simulink model "PV_grid_connected_Inverter"  (R2022b)
settings: Solver=ode23tb  StartTime=0.0  StopTime=2  FixedStep=Ts_Power  RelTol=1e-4
PreLoadFcn:
  | Ts_Power=50e-6;
  | Ts_Control=100e-6;
InitFcn:
  | Ts_Power=50e-6;
  | Ts_Control=100e-6;
undefined symbols (not defined in the file): sigbuilder_block
libraries: spsIGBTDiodeLib x7, spsSeriesRLCBranchLib x3, spsThreePhaseSeriesRLCBranchLib x1, spsThreePhaseSourceLib x1, slpidlib x1, spsPLL3phLib x1, spsabctodq0Lib x1, spsdq0toabcLib x1, spsDiodeLib x1, spsGroundLib x1, spsMeanLib x1, spsPower3phInstantaneousLib x1
Description:
  | Copyright 2008-2017 The MathWorks, Inc.
settings Model: Creator=MathWorks  LastModifiedBy=mohua
settings SolverCC: SolverJacobianMethodControl=FullAnalytical  ZeroCrossAlgorithm=Adaptive  AlgebraicLoopSolver=TrustRegion
settings DataIOCC: LimitDataPoints=on  SaveFormat=Array  SignalLoggingSaveFormat=ModelDataLogs  ReturnWorkspaceOutputs=off
settings OptimizationCC: ExpressionDepthLimit=2147483647  LifeSpan=inf
settings DebuggingCC: UnderspecifiedInitializationDetection=Classic  MergeDetectMultiDrivingBlocksExec=none  SolverPrmCheckMsg=warning  FcnCallInpInsideContextMsg=warning  UnconnectedInputMsg=warning  UnconnectedOutputMsg=warning  UnconnectedLineMsg=warning  StateNameClashWarn=warning  SFUnexpectedBacktrackingDiag=warning  SFNoUnconditionalDefaultTransitionDiag=warning  SFExecutionAtInitializationDiag=none  SFMachineParentedDataDiag=warning  ArithmeticOperatorsInVariantConditions=warning
settings HardwareCC: ProdBitPerPointer=32  ProdBitPerSizeT=32  ProdBitPerPtrDiffT=32  ProdLargestAtomicFloat=None  ProdIntDivRoundTo=Undefined  ProdEndianess=Unspecified  ProdWordSize=32  ProdHWDeviceType=32-bit Generic
settings ModelReferenceCC: EnableRefExpFcnMdlSchedulingChecks=on  PropagateSignalLabelsOutOfModel=off
settings SFSimCC: SimUseLocalCustomCode=off  CustomCodeUndefinedFunction=UseInterfaceOnly
settings RTWCC: RTWUseLocalCustomCode=off
settings CodeAppCC: StateflowObjectComments=on
settings GRTTargetCC: TargetLangStandard=C89/C90 (ANSI)  CombineOutputUpdateFcns=off  GRTInterface=on
settings ConfigComp: CovMetricSettings=dw  CovSaveCumulativeToWorkspaceVar=on  CovSaveSingleToWorkspaceVar=on  CovExternalEMLEnable=off  CovSFcnEnable=off
settings SimscapeCC: SimscapeNormalizeSystem=off

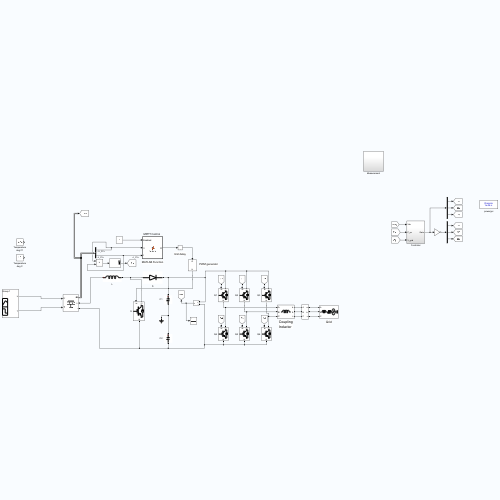
[thumbnail: Simulink's stored preview of the top-level diagram]
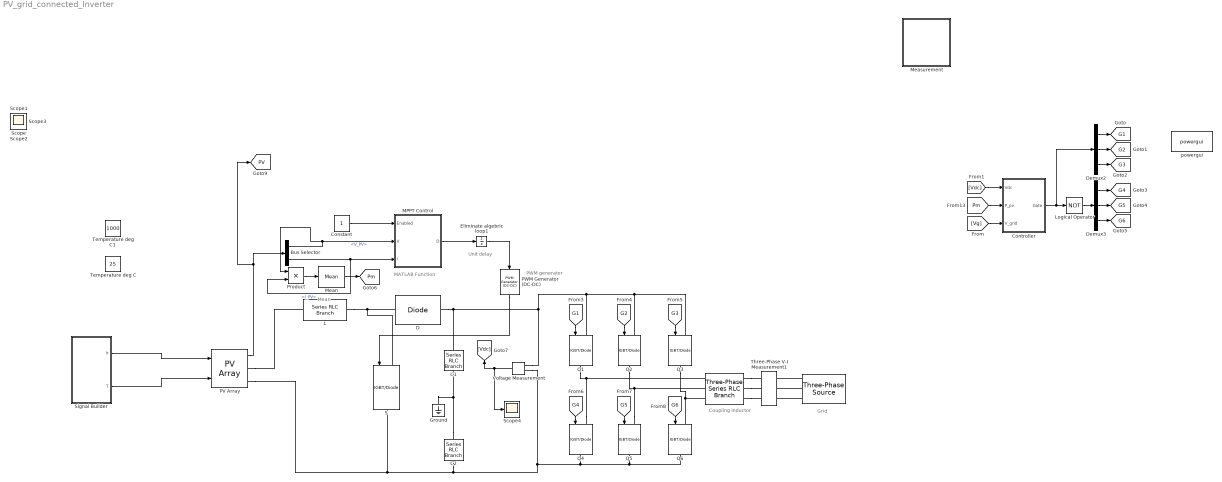
== system PV_grid_connected_Inverter ==
  note: Grid
  note: Coupling
      | Inductor
  note: MATLAB Function
  note: Mean
  note: PWM generator
  note: Unit delay
  " " : spsThreePhaseSeriesRLCBranchLib/Three-Phase Series RLC Branch  LConnTagsString=A|B|C  RConnTagsString=A|B|C  BranchType=L  Resistance=0.09  Inductance=0.28e-3  Capacitance=1e-6  Measurements=None
  "  " : spsThreePhaseSourceLib/Three-Phase Source  InternalConnection=Yg  VoltagePhases=off  Voltage=400  PhaseAngle=0  Voltage_phases=[25e3 25e3 25e3]/sqrt(3)  PhaseAngles_phases=[0 -120 +120]  Frequency=50  NonIdealSource=on  SpecifyImpedance=on  Resistance=0.8929  Inductance=16.58e-3  ShortCircuitLevel=100e6  BaseVoltage=400  XRratio=10  BusType=swing  Pref=0  Qref=0  Prefabc=[10e3, 10e3, 10e3]  Qrefabc=[0, 0, 0]  Qmin=-inf  Qmax=inf
  Bus Selector : BusSelector  OutputSignals=V_PV,I_PV
  C1 : spsSeriesRLCBranchLib/Series RLC Branch  LConnTagsString=__new0  RConnTagsString=__new0  BranchType=C  Resistance=1  Inductance=1e-3  SetiL0=off  InitialCurrent=0  Capacitance=4700e-6  Setx0=on  InitialVoltage=350  Measurements=None
  C2 : spsSeriesRLCBranchLib/Series RLC Branch  LConnTagsString=__new0  RConnTagsString=__new0  BranchType=C  Resistance=1  Inductance=1e-3  SetiL0=off  InitialCurrent=0  Capacitance=4700e-6  Setx0=on  InitialVoltage=350  Measurements=None
  Constant : Constant
  Controller : Subsystem
  D : spsDiodeLib/Diode  Ron=0.001  Lon=0  Vf=0.8  IC=0  UseSnubber=0  Rs=inf  Cs=250e-9  Measurements=off
  Demux2 : Demux  Outputs=3
  Demux3 : Demux  Outputs=3
  Eliminate algebric loop1 : UnitDelay  InitialCondition=0.485  SampleTime=Ts_Control  HasFrameUpgradeWarning=on
  Ground : spsGroundLib/Ground  LConnTagsString=a
  L : spsSeriesRLCBranchLib/Series RLC Branch  LConnTagsString=__new0  RConnTagsString=__new0  BranchType=L  Resistance=0.001  Inductance=4e-3  SetiL0=off  InitialCurrent=0  Capacitance=1e-6  Setx0=off  InitialVoltage=0  Measurements=None
  Logical Operator : Logic  Operator=NOT  IconShape=distinctive  AllPortsSameDT=off  OutDataTypeStr=boolean
  "MPPT Control  " : MATLAB Function  TreatAsAtomicUnit=on
  Mean : spsMeanLib/Mean  Freq=50  Vinit=0  Ts=0
  Measurement : Subsystem
  PV Array : spsPVArrayLib/PV Array  Npar=64  Nser=5  PlotType=array @ 1000 W/m2 & specified temperatures  S_vec="[ 1000  500  100 ]"  Temp_C_vec="[ 45 25  ]"  ModuleName=SunPower SPR-315E-WHT-D  PlotWhenSelected=off  Pm=315.072  Ncell=96  Voc=64.6  Isc=6.14  Vm=54.7  Im=5.76  beta_Voc_pc=-0.2727  alpha_Isc_pc=0.061743  beta_Voc=-0.17616  alpha_Isc=0.003791  IL=6.1461  I0=6.5067e-12  nI=0.95071  Rsh=430.0666  Rs=0.43041  RobustModel=off  RobustCellTemperature=25  BAL=off  Tc=1e-6  Tfilter=5e-5
  PWM Generator (DC-DC) : spsPWMGeneratorDCDCLib/PWM Generator (DC-DC)  Fsw=5000  Ts=0
  Product : Product
  Q{1..6} (6 alike) : spsIGBTDiodeLib/IGBT//Diode  Ron=1e-3  Rs=1e5  Cs=inf  Measurements=off
  S : spsIGBTDiodeLib/IGBT//Diode  Ron=1e-3  Rs=1e5  Cs=inf  Measurements=off
  Scope{,1..4} (5 alike) : Scope
  Signal Builder : Subsystem  Tag=STV Subsys  LoadFcn=sigbuilder_block('load');  StartFcn=sigbuilder_block('start');  StopFcn=sigbuilder_block('stop');  ClipboardFcn=sigbuilder_block('clipboard');  mask(Sigbuilder block){tuvar=[0:10]}
      mask help: Simulink:masks:SigbuilderBlock_MD
      mask init:
      | if ~strcmp(get_param(bdroot(gcbh),'SimulationStatus'),'stopped') tuvar = sigbuilder_block('maskInit'); end
      settings: CopyFcn=sigbuilder_block('copy');  DeleteFcn=sigbuilder_block('delete');  ModelCloseFcn=sigbuilder_block('modelClose');  PreSaveFcn=sigbuilder_block('preSave');  PauseFcn=sigbuilder_block('pause');  ContinueFcn=sigbuilder_block('continue');  NameChangeFcn=sigbuilder_block('namechange');  OpenFcn=sigbuilder_block('open',[441.6 157.2 550.8 400.2 ]);  CloseFcn=sigbuilder_block('close');
      mask Display: plot(0, 0, 100, 100,[2, 2, 32, 32, 2], [68, 8, 8, 68, 68],[32, 2], [38, 38], [32, 19, 2],[53, 60, 44], [32, 17, 17, 2],[16, 16, 31, 31]);txt = getActiveGroup(gcbh);text(2, 100, txt,'verticalAlignment', 'top');
  Temperature deg C : Constant  Value=25
  Temperature deg C1 : Constant  Value=1000
  Three-Phase V-I Measurement1 : spsThreePhaseVIMeasurementLib/Three-Phase V-I Measurement  VoltageMeasurement=phase-to-ground  SetLabelV=on  LabelV=Vg  Vpu=off  VpuLL=off  CurrentMeasurement=yes  SetLabelI=on  LabelI=Icom  Ipu=off  Pbase=100e6  Vbase=500e3  OutputType=Complex  PhasorSimulation=off  PSBequivalent=0
  Voltage Measurement : spsVoltageMeasurementLib/Voltage Measurement  PhasorSimulation=off  OutputType=Complex  PSBequivalent=0
  powergui : spspowerguiLib/powergui  Priority=1  SimulationMode=Discrete  SampleTime=1e-6  frequency=60  Iterations=50  frequencyindice=0  Pbase=100e6  ErrMax=1e-4  UnitsV=kV  UnitsW=MW  buscounter=0  FunctionMessages=off  echomessages=off  EnableUseOfTLC=off  CurrentSourceSwitches=off  DisableSnubberDevices=off  DisableRonSwitches=off  DisableVfSwitches=off  DisplayEquations=off  AutomaticDiscreteSolvers=off  SolverType=Tustin/Backward Euler (TBE)  Interpol=off  ExternalGateDelay=off  methode=off  Ts=100  x0status=blocks  SPID=on  SwTol=0  HookPort=off  NonlinearTolerance=1e-4  nMaxIteration=100  ContinueOnMaxIteration=off  RestoreLinks=warning  ResistiveCurrentMeasurement=off  Frange=[0:2:500]  Ylog=off  Xlog=on  ShowGrid=off  save=off  variable=ZData  structure=0  ZoomFFT=off  StartTime=0.0  cycles=1  DisplayStyle=1  fundamental=60  FreqAxis=off  MaxFrequency=1000  frequencyindicesteady=1  RmsSteady=1  display=off
  tag scope: G1=global, G2=global, G3=global, G4=global, G5=global, G6=global, PV=global, Pm=global
  wires:
  PV Array/1 -> [PV], Bus Selector/1
  Bus Selector/2 -> Product/2, "MPPT Control  "/3(I)  "<I_PV>"
  "MPPT Control  "/1(D) -> Eliminate algebric loop1/1
  PWM Generator (DC-DC)/1 -> S/1
  Product/1 -> Mean/1
  [G5] -> Q5/1
  [G4] -> Q4/1
  Demux2/2 -> [G2]
  Demux3/2 -> [G5]
  [G1] -> Q1/1
  Demux3/1 -> [G4]
  Demux2/3 -> [G3]
  Demux2/1 -> [G1]
  [G3] -> Q3/1
  [G2] -> Q2/1
  Logical Operator/1 -> Demux3/1
  [G6] -> Q6/1
  Demux3/3 -> [G6]
  Mean/1 -> [Pm]
  Controller/1(Gate) -> Logical Operator/1, Demux2/1
  [Pm] -> Controller/2(P_pv)
  [Vg] -> Controller/3(V_grid)
  Eliminate algebric loop1/1 -> PWM Generator (DC-DC)/1
  Bus Selector/1 -> "MPPT Control  "/2(V), Product/1  "<V_PV>"
  Constant/1 -> "MPPT Control  "/1(Enabled)
  Voltage Measurement/1 -> Scope4/1, [Vdc]
  [Vdc] -> Controller/1(Vdc)
  Signal Builder/1(Ir) -> PV Array/1
  Signal Builder/2(T) -> PV Array/2
  connections:
  L/RConn1 -- S/LConn1 -- D/LConn1
  PV Array/RConn1 -- L/LConn1
  PV Array/RConn2 -- Q6/RConn1 -- Q5/RConn1 -- Q4/RConn1 -- Voltage Measurement/LConn2 -- C2/RConn1 -- S/RConn1
  D/RConn1 -- C1/LConn1 -- Q1/LConn1 -- Q2/LConn1 -- Q3/LConn1 -- Voltage Measurement/LConn1
  Q3/RConn1 -- " "/LConn3 -- Q6/LConn1
  C2/LConn1 -- Ground/LConn1 -- C1/RConn1
  Q4/LConn1 -- Q1/RConn1 -- " "/LConn1
  Q5/LConn1 -- Q2/RConn1 -- " "/LConn2
  " "/RConn3 -- Three-Phase V-I Measurement1/LConn3
  " "/RConn1 -- Three-Phase V-I Measurement1/LConn1
  " "/RConn2 -- Three-Phase V-I Measurement1/LConn2
  "  "/RConn1 -- Three-Phase V-I Measurement1/RConn1
  "  "/RConn2 -- Three-Phase V-I Measurement1/RConn2
  "  "/RConn3 -- Three-Phase V-I Measurement1/RConn3

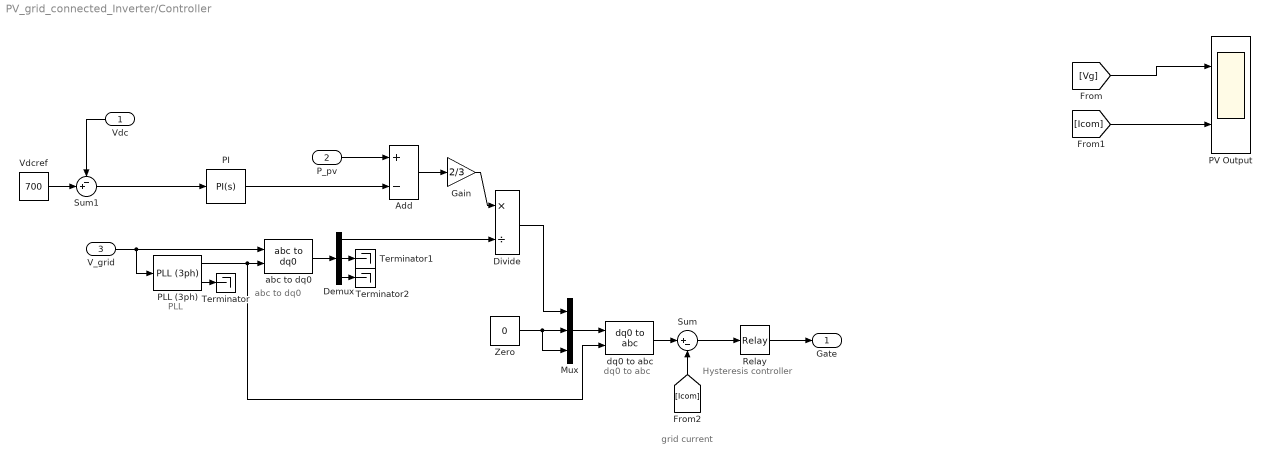
== system PV_grid_connected_Inverter/Controller ==
  note: dq0 to abc
  note: abc to dq0
  note: PLL
  note: Hysteresis controller
  note: grid current
  Vdc : Inport
  P_pv : Inport  Port=2
  V_grid : Inport  Port=3
  Add : Sum  Inputs=+-
  Demux : Demux  Outputs=3
  Divide : Product  Inputs=*/
  Gain : Gain  Gain=2/3
  Mux : Mux  Inputs=3
  PI : slpidlib/PID Controller  Controller=PI  Form=Parallel  TimeDomain=Continuous-time  UseExternalTs=off  SampleTime=-1  IntegratorMethod=Forward Euler  FilterMethod=Forward Euler  ControllerParametersSource=internal  P=112  I=735  UseKiTs=off  D=0  N=100  UseFilter=on  TunerSelectOption=Transfer Function Based (PID Tuner App)  InitialConditionSource=internal  InitialConditionForIntegrator=0  InitialConditionForFilter=0  DifferentiatorICPrevScaledInput=0  ExternalReset=none  TrackingMode=off  Kt=1  LimitOutput=off  SatLimitsSource=internal  UpperSaturationLimit=inf  LowerSaturationLimit=-inf  LinearizeAsGain=on  AntiWindupMode=none  Kb=1  LimitIntegrator=off  UpperIntegratorSaturationLimit=inf  LowerIntegratorSaturationLimit=-inf  POutMin=[]  POutMax=[]  IOutMin=[]  IOutMax=[]  DOutMin=[]  DOutMax=[]  NOutMin=[]  NOutMax=[]  SumOutMin=[]  SumOutMax=[]  SaturationOutMin=[]  SaturationOutMax=[]  PParamMin=[]  PParamMax=[]  IParamMin=[]  IParamMax=[]  DParamMin=[]  DParamMax=[]  NParamMin=[]  NParamMax=[]  KbParamMin=[]  KbParamMax=[]  KtParamMin=[]  KtParamMax=[]  KbOutMin=[]  KbOutMax=[]  KtOutMin=[]  KtOutMax=[]  IntegratorOutMin=[]  IntegratorOutMax=[]  FilterOutMin=[]  FilterOutMax=[]  SumI1OutMin=[]  SumI1OutMax=[]  SumI2OutMin=[]  SumI2OutMax=[]  SumI3OutMin=[]  SumI3OutMax=[]  SumI4OutMin=[]  SumI4OutMax=[]  SumDOutMin=[]  SumDOutMax=[]  DifferentiatorOutMin=[]  DifferentiatorOutMax=[]  FilterDiffOutCoefMin=[]  FilterDiffOutCoefMax=[]  ReciprocalOutMin=[]  ReciprocalOutMax=[]  SumDenOutMin=[]  SumDenOutMax=[]  SumNumOutMin=[]  SumNumOutMax=[]  DivideOutMin=[]  DivideOutMax=[]  UdiffTsProdOutMin=[]  UdiffTsProdOutMax=[]  NTsProdOutMin=[]  NTsProdOutMax=[]  UintegralTsProdOutMin=[]  UintegralTsProdOutMax=[]  UngainTsProdOutMin=[]  UngainTsProdOutMax=[]  ClampingZeroOutDataTypeStr=Inherit: Inherit via back propagation  ClampingZeroOutMin=[]  ClampingZeroOutMax=[]  FilterDenConstantOutDataTypeStr=Inherit: Inherit via back propagation  FilterDenConstantOutMin=[]  FilterDenConstantOutMax=[]  PCopyOutDataTypeStr=Inherit: Inherit via back propagation  PCopyOutMin=[]  PCopyOutMax=[]  NCopyOutDataTypeStr=Inherit: Inherit via back propagation  NCopyOutMin=[]  NCopyOutMax=[]  IntegratorContinuousStateAttributes=''  IntegratorStateMustResolveToSignalObject=off  IntegratorRTWStateStorageClass=Auto  FilterContinuousStateAttributes=''  FilterStateMustResolveToSignalObject=off  FilterRTWStateStorageClass=Auto  ParallelPVariant=InternalParameters  IdealPVariant=Disabled  IVariant=InternalParameters  DVariant=Disabled  IntegratorVariant=Continuous  SatVariant=Disabled  AWVariant=Passthrough  PCopyVariant=Disabled  TRVariant=Disabled  FdbkBlocksVariant=Forward  IdealPFdbkVariant=Disabled  SatFdbkVariant=Disabled  DerivativeFilterVariant=Disabled  NVariant=Disabled  NCopyVariant=Disabled_SignalSpec  FilterICVariant=Disabled  IntegratorICVariant=InternalICs  ExternalResetVariant=Disabled  TRSumVariant=Passthrough  SumFdbkVariant=Disabled  SumVariant=Sum_PI  TsampFilterVariant=InternalTs  TsampNgainVariant=Passthrough  TsampIntegralVariant=Passthrough  ExternalSaturationOutDataTypeStr=Inherit: Same as second input
  PLL (3ph) : spsPLL3phLib/PLL (3ph)  Fmin=45  Par_Init=[0, 60]  ParK=[180, 3200, 1]  TcD=1e-4  MaxRateChangeFreq=12  FilterCutOffFreq=25  Ts=0  AGC=on
  PV Output : Scope  NumInputPorts=2
  Relay : Relay  OnSwitchValue=0.1  OffSwitchValue=-0.1
  Sum : Sum  Inputs=|+-
  Sum1 : Sum  Inputs=-+|
  Terminator : Terminator
  Terminator1 : Terminator
  Terminator2 : Terminator
  Vdcref : Constant  Value=700
  Zero : Constant  Value=0
  abc to dq0 : spsabctodq0Lib/abc to dq0  Alignment=90 degrees behind phase A axis
  dq0 to abc : spsdq0toabcLib/dq0 to abc  Alignment=90 degrees behind phase A axis
  Gate : Outport
  wires:
  Add/1 -> Gain/1
  Sum1/1 -> PI/1
  Vdc/1 -> Sum1/1
  dq0 to abc/1 -> Sum/1
  PI/1 -> Add/2
  Relay/1 -> Gate/1
  Mux/1 -> dq0 to abc/1
  abc to dq0/1 -> Demux/1
  P_pv/1 -> Add/1
  Gain/1 -> Divide/1
  V_grid/1 -> abc to dq0/1, PLL (3ph)/1
  Divide/1 -> Mux/1
  PLL (3ph)/1 -> Terminator/1
  Zero/1 -> Mux/3, Mux/2
  Demux/2 -> Terminator1/1
  Demux/3 -> Terminator2/1
  Demux/1 -> Divide/2
  PLL (3ph)/2 -> dq0 to abc/2, abc to dq0/2
  Sum/1 -> Relay/1
  [Icom] -> Sum/2
  Vdcref/1 -> Sum1/2
  [Icom] -> PV Output/2
  [Vg] -> PV Output/1

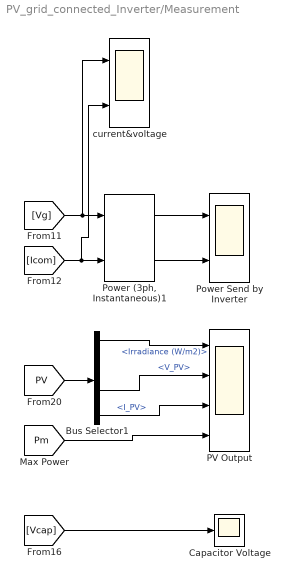
== system PV_grid_connected_Inverter/Measurement ==
  Bus Selector1 : BusSelector  OutputSignals=Irradiance (W/m2),Temperature (deg C),V_PV,I_PV
  Capacitor Voltage : Scope
  PV Output : Scope  NumInputPorts=4
  "Power (3ph, Instantaneous)1" : spsPower3phInstantaneousLib/Power (3ph, Instantaneous)
  Power Send by Inverter : Scope  NumInputPorts=2
  current&voltage : Scope  NumInputPorts=2
  wires:
  [Vg] -> current&voltage/1, "Power (3ph, Instantaneous)1"/1
  [Icom] -> current&voltage/2, "Power (3ph, Instantaneous)1"/2
  "Power (3ph, Instantaneous)1"/1 -> Power Send by Inverter/1
  "Power (3ph, Instantaneous)1"/2 -> Power Send by Inverter/2
  Bus Selector1/3 -> PV Output/2  "<V_PV>"
  [Pm] -> PV Output/4
  Bus Selector1/1 -> PV Output/1  "<Irradiance (W/m2)>"
  [PV] -> Bus Selector1/1
  [Vcap] -> Capacitor Voltage/1
  Bus Selector1/4 -> PV Output/3  "<I_PV>"

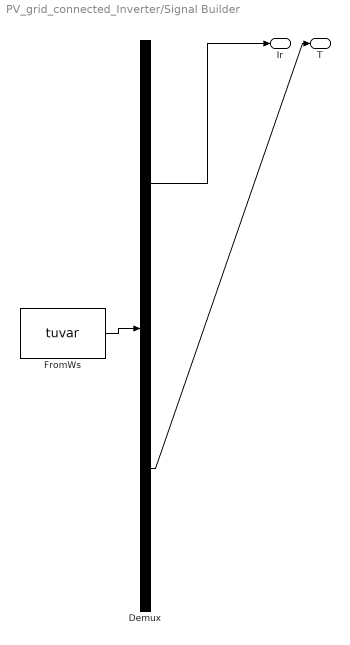
== system PV_grid_connected_Inverter/Signal Builder ==
  Demux : Demux  Tag=STV Demux  Outputs=2
      settings: DisplayOption=none
  FromWs : FromWorkspace  Tag=STV FromWs  VariableName=tuvar
      SigBuilderData=|
      | common.afterFinalStr = 'Extrapolate'
      | common.sampleTime = 0
      | dataSet.timeRange = [0 10]
      | dataSet.name = 'Group 1'
      | sbobj.Groups.Name = 'Group 1'
      | sbobj.Groups.Signals(1).Name = 'Ir'
      | sbobj.Groups.Signals(1).XData = [0 0.96 0.96 1.32 1.32 6 10]
      | sbobj.Groups.Signals(1).YData = [1000 1000 900 902 1002 998 1000]
      | sbobj.Groups.Signals(2).Name = 'T'
      | sbobj.Groups.Signals(2).XData = [0 0.98 0.98 1.6 1.6 4 6 10]
      | sbobj.Groups.Signals(2).YData = [24 24 30.1 29.9 23.9 24 24 24]
  Ir : Outport  Tag=STV Outport
  T : Outport  Tag=STV Outport  Port=2
  wires:
  Demux/1 -> Ir/1
  FromWs/1 -> Demux/1
  Demux/2 -> T/1

== matlab function PV_grid_connected_Inverter/MPPT Control   ==
  settings: updateMethod=DISCRETE  sampleTime=Ts_Control
  data: Enabled input; V input =V; I input; D output
function D  = PandO(Enabled, V, I)

Dinit = 0.62;  %Initial value for D output
Dmax = 0.8;   %Maximum value for D
Dmin = 0.2;   %Minimum value for D
deltaD = 2e-4; %Increment value used to increase/decrease the duty cycle D

persistent Vold Pold Dold;

dataType = 'double';

if isempty(Vold)
    Vold=0;
    Pold=0;
    Dold=Dinit;
end
P= V*I;
dV= V - Vold;
dP= P - Pold;

if dP ~= 0 & Enabled ~=0
    if dP < 0
        if dV < 0
            D = Dold - deltaD;
        else
            D = Dold + deltaD;
        end
    else
        if dV < 0
            D = Dold + deltaD;
        else
            D = Dold - deltaD;
        end    
    end
else D=Dold;
end

if D >= Dmax | D<= Dmin
    D=Dold;
end

Dold=D;
Vold=V;
Pold=P;
